simulink model "Schemi_Simulink_Tesina_Controlli"  (R2023b)
settings: Solver=VariableStepAuto  StartTime=0.0  StopTime=50  RelTol=1e-3
undefined symbols (not defined in the file): A, A_Kal, A_obs, Ar, B, B_Kal, B_obs, Br, C, C_Kal, C_obs, Cr, D, D_Kal, D_obs, Dr, Fi, Fr, Ki, Kr, Tc
libraries: simulink x7
settings Model: Creator=emman  LastModifiedBy=emman

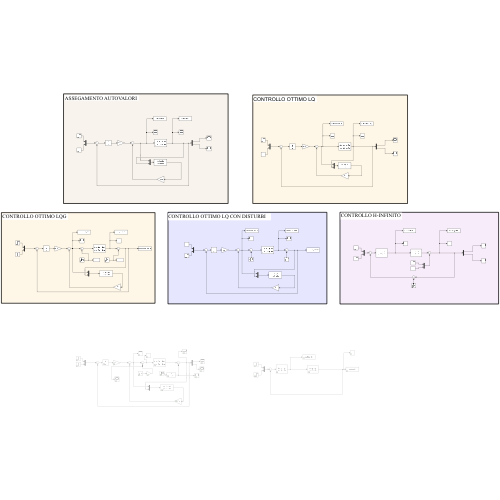
[thumbnail: Simulink's stored preview of the top-level diagram]
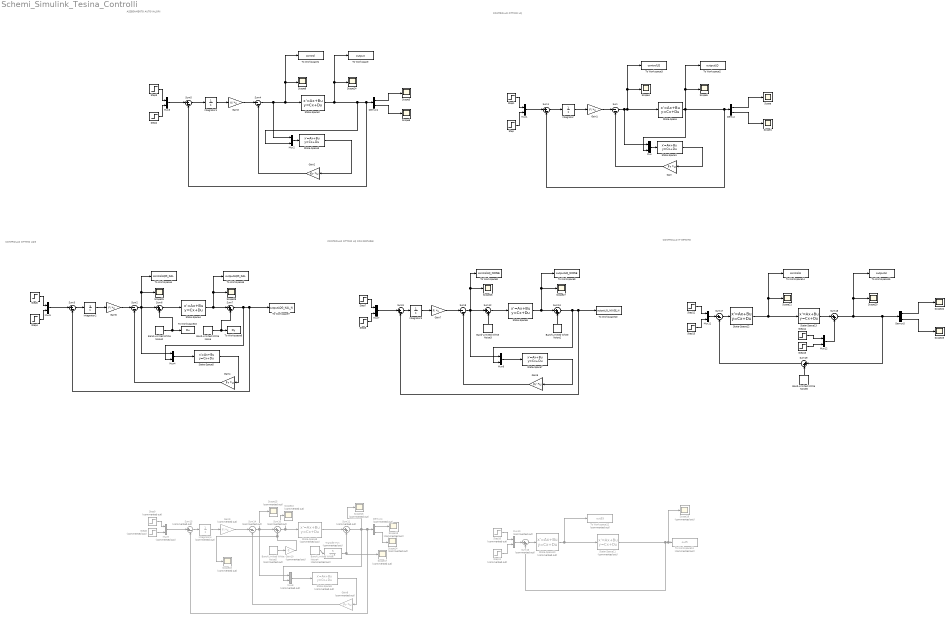
== system Schemi_Simulink_Tesina_Controlli ==
  note: CONTROLLO H-INFINITO
  note: CONTROLLO OTTIMO LQG
  note: CONTROLLO OTTIMO LQ CON DISTURBI
  note: CONTROLLO OTTIMO LQ
  note: ASSEGAMENTO AUTOVALORI
  Band-Limited White Noise : simulink/Sources/Band-Limited White Noise  Cov=NoisePower  Ts=Tc  seed=[23341]
  Band-Limited White Noise1 : simulink/Sources/Band-Limited White Noise  Cov=NoisePower  Ts=Tc  seed=[23341]
  Band-Limited White Noise2 : simulink/Sources/Band-Limited White Noise  Cov=Qnoise  Ts=Tc  seed=[23341]
  Band-Limited White Noise3 : simulink/Sources/Band-Limited White Noise  Cov=Qnoise  Ts=Tc  seed=[23341]
  Band-Limited White Noise4 : simulink/Sources/Band-Limited White Noise  Commented=on  Cov=NoisePower  Ts=Tc  seed=[23341]
  Band-Limited White Noise5 : simulink/Sources/Band-Limited White Noise  Commented=on  Cov=Qnoise  Ts=Tc  seed=[23341]
  Band-Limited White Noise6 : simulink/Sources/Band-Limited White Noise  Cov=NoisePower  Ts=Tc  seed=[23341]
  Demux : Demux  Outputs=2
  Demux1 : Demux  Outputs=2
  Demux4 : Demux  Commented=on  Outputs=2
  Demux5 : Demux  Outputs=2
  Gain : Gain  Gain=Fr  Multiplication=Matrix(K*u)
  Gain1 : Gain  Gain=Fi  Multiplication=Matrix(K*u)
  Gain10 : Gain  Commented=on  Gain=0
  Gain2 : Gain  Gain=Kr  Multiplication=Matrix(K*u)
  Gain3 : Gain  Gain=Ki  Multiplication=Matrix(K*u)
  Gain4 : Gain  Gain=Fr  Multiplication=Matrix(K*u)
  Gain5 : Gain  Gain=Fi  Multiplication=Matrix(K*u)
  Gain6 : Gain  Gain=Fr  Multiplication=Matrix(K*u)
  Gain7 : Gain  Gain=Fi  Multiplication=Matrix(K*u)
  Gain8 : Gain  Commented=on  Gain=Fr  Multiplication=Matrix(K*u)
  Gain9 : Gain  Commented=on  Gain=Fi  Multiplication=Matrix(K*u)
  Integrator{,1..3} (4 alike) : Integrator
  Integrator4 : Integrator  Commented=on
  Mux{,1..7,11..12} (10 alike) : Mux  Inputs=2
  Mux10 : Mux  Commented=on  Inputs=2
  Mux8 : Mux  Commented=on  Inputs=2
  Mux9 : Mux  Commented=on  Inputs=2
  Scope{,1,3..6,8,20..28} (16 alike) : Scope
  Scope{10,13..19} (8 alike) : Scope  Commented=on
  State-Space{,2,4,6} (4 alike) : StateSpace  A=A  B=B  C=C  D=D  InitialCondition=0  ParameterTunability=Unconstrained
  State-Space1 : StateSpace  A=A_obs  B=B_obs  C=C_obs  D=D_obs  InitialCondition=0
  State-Space10 : StateSpace  Commented=on  A=Ar  B=Br  C=Cr  D=Dr  InitialCondition=0
  State-Space11 : StateSpace  Commented=on  A=A  B=B  C=C  D=D  InitialCondition=0
  State-Space12 : StateSpace  A=Ar  B=Br  C=Cr  D=Dr  InitialCondition=0
  State-Space13 : StateSpace  A=A  B=B  C=C  D=D  InitialCondition=0
  State-Space3 : StateSpace  A=A_obs  B=B_obs  C=C_obs  D=D_obs  InitialCondition=0
  State-Space5 : StateSpace  A=A_Kal  B=B_Kal  C=C_Kal  D=D_Kal  InitialCondition=0
  State-Space7 : StateSpace  A=A_obs  B=B_obs  C=C_obs  D=D_obs  InitialCondition=0
  State-Space8 : StateSpace  Commented=on  A=A  B=B  C=C  D=D  InitialCondition=0  ParameterTunability=Unconstrained
  State-Space9 : StateSpace  Commented=on  A=A_obs  B=B_obs  C=C_obs  D=D_obs  InitialCondition=0
  Step{,2,4,6,13} (5 alike) : Step  Time=0  After=2.5  SampleTime=0
  Step{1,3,5,7,12} (5 alike) : Step  Time=0  After=2  SampleTime=0
  Step10 : Step  Commented=on  Time=0  After=2  SampleTime=0
  Step11 : Step  Commented=on  Time=0  After=2.5  SampleTime=0
  Step14 : Step  Time=0  After=0.5  SampleTime=0
  Step15 : Step  Time=0  After=0.5  SampleTime=0
  Step8 : Step  Commented=on  Time=0  After=2.5  SampleTime=0
  Step9 : Step  Commented=on  Time=0  After=2  SampleTime=0
  Sum{,2,4,8} (4 alike) : Sum  Inputs=|--
  Sum{1,3,5,9,17} (5 alike) : Sum  Inputs=|+-
  Sum10 : Sum  Commented=on  Inputs=|++
  Sum11 : Sum  Commented=on  Inputs=|++
  Sum{6..7,12..13,18..19} (6 alike) : Sum  Inputs=|++
  Sum14 : Sum  Commented=on  Inputs=|--
  Sum15 : Sum  Commented=on  Inputs=|+-
  Sum16 : Sum  Commented=on  Inputs=|+-
  To Workspace : ToWorkspace  VariableName=output  SaveFormat=Structure With Time  SampleTime=-1
  To Workspace1 : ToWorkspace  VariableName=control  SaveFormat=Structure With Time  SampleTime=-1
  To Workspace10 : ToWorkspace  VariableName=outputLQ_NOISE_N  SaveFormat=Structure With Time  SampleTime=-1
  To Workspace12 : ToWorkspace  Commented=on  VariableName=out55  SaveFormat=Structure With Time  SampleTime=-1
  To Workspace13 : ToWorkspace  Commented=on  VariableName=out5  SaveFormat=Structure With Time  SampleTime=-1
  To Workspace14 : ToWorkspace  VariableName=controlH  SaveFormat=Structure With Time  SampleTime=-1
  To Workspace15 : ToWorkspace  VariableName=outputH  SaveFormat=Structure With Time  SampleTime=-1
  To Workspace16 : ToWorkspace  VariableName=Du  SaveFormat=Structure With Time  SampleTime=-1
  To Workspace2 : ToWorkspace  VariableName=outputLQ  SaveFormat=Structure With Time  SampleTime=-1
  To Workspace3 : ToWorkspace  VariableName=controlLQ  SaveFormat=Structure With Time  SampleTime=-1
  To Workspace4 : ToWorkspace  VariableName=controlLQG_KAL  SaveFormat=Structure With Time  SampleTime=-1
  To Workspace5 : ToWorkspace  VariableName=outputLQG_KAL  SaveFormat=Structure With Time  SampleTime=-1
  To Workspace6 : ToWorkspace  VariableName=Dy  SaveFormat=Structure With Time  SampleTime=-1
  To Workspace7 : ToWorkspace  VariableName=outputLQG_KAL_N  SaveFormat=Structure With Time  SampleTime=-1
  To Workspace8 : ToWorkspace  VariableName=controlLQ_NOISE  SaveFormat=Structure With Time  SampleTime=-1
  To Workspace9 : ToWorkspace  VariableName=outputLQ_NOISE  SaveFormat=Structure With Time  SampleTime=-1
  Transfer Fcn : TransferFcn  Commented=on  Numerator=[5]  Denominator=[1 5]
  wires:
  Sum4/1 -> To Workspace1/1, Scope8/1, State-Space2/1, Mux2/1
  Integrator1/1 -> Gain3/1
  State-Space2/1 -> To Workspace/1, Scope24/1, Sum5/2, Demux1/1, Mux2/2
  State-Space3/1 -> Gain2/1
  Gain2/1 -> Sum4/2
  Demux1/1 -> Scope3/1
  Mux2/1 -> State-Space3/1
  Mux3/1 -> Sum5/1
  Demux1/2 -> Scope6/1
  Gain3/1 -> Sum4/1
  Step2/1 -> Mux3/2
  Sum5/1 -> Integrator1/1
  Step3/1 -> Mux3/1
  Gain1/1 -> Sum/1
  Sum/1 -> Scope4/1, To Workspace3/1, State-Space/1, Mux/1
  State-Space1/1 -> Gain/1
  Step/1 -> Mux1/2
  Mux1/1 -> Sum1/1
  Gain/1 -> Sum/2
  Sum1/1 -> Integrator/1
  State-Space/1 -> To Workspace2/1, Scope5/1, Sum1/2, Demux/1, Mux/2
  Step1/1 -> Mux1/1
  Mux/1 -> State-Space1/1
  Integrator/1 -> Gain1/1
  Demux/1 -> Scope/1
  Demux/2 -> Scope1/1
  Gain4/1 -> Sum2/2
  Step4/1 -> Mux5/2
  Sum3/1 -> Integrator2/1
  Step7/1 -> Mux7/1
  Integrator3/1 -> Gain7/1
  Sum8/1 -> Scope26/1, To Workspace8/1, Mux6/1, Sum12/1
  Sum2/1 -> Scope25/1, To Workspace4/1, Mux4/1, Sum6/1
  Band-Limited White Noise/1 -> Sum7/2, To Workspace6/1
  Sum6/1 -> State-Space4/1
  Band-Limited White Noise2/1 -> Sum6/2, To Workspace16/1
  Gain6/1 -> Sum8/2
  Band-Limited White Noise5/1 -> Gain10/1
  Gain10/1 -> Scope18/1, Sum10/2
  Sum14/1 -> Scope15/1, Mux8/1, Sum10/1
  State-Space8/1 -> Sum11/1
  Sum11/1 -> Scope16/1, Mux8/2, Sum15/2, Demux4/1
  Sum7/1 -> To Workspace7/1, Sum3/2, Mux4/2
  State-Space5/1 -> Gain4/1
  State-Space6/1 -> Scope27/1, To Workspace9/1, Sum13/1
  Gain5/1 -> Sum2/1
  Step8/1 -> Mux9/2
  Mux5/1 -> Sum3/1
  Gain8/1 -> Sum14/2
  Gain7/1 -> Sum8/1
  Gain9/1 -> Sum14/1
  Mux8/1 -> State-Space9/1
  Sum9/1 -> Integrator3/1
  Integrator2/1 -> Gain5/1
  Demux4/2 -> Scope14/1
  Mux9/1 -> Sum15/1
  Step9/1 -> Mux9/1
  Sum13/1 -> Mux6/2, To Workspace10/1, Sum9/2
  Band-Limited White Noise4/1 -> Transfer Fcn/1
  Integrator4/1 -> Gain9/1
  Mux6/1 -> State-Space7/1
  Transfer Fcn/1 -> Scope17/1, Sum11/2
  Sum12/1 -> State-Space6/1
  Sum10/1 -> Scope10/1, State-Space8/1
  Step6/1 -> Mux7/2
  State-Space9/1 -> Gain8/1
  Mux4/1 -> State-Space5/1
  Mux7/1 -> Sum9/1
  Sum15/1 -> Integrator4/1
  State-Space4/1 -> Scope28/1, To Workspace5/1, Sum7/1
  Step5/1 -> Mux5/1
  State-Space7/1 -> Gain6/1
  Demux4/1 -> Scope13/1
  Step12/1 -> Mux11/1
  Sum18/1 -> Sum19/1, Demux5/1, Scope20/1, To Workspace15/1
  State-Space13/1 -> Sum18/1
  Mux12/1 -> Sum18/2
  Sum17/1 -> State-Space12/1
  Step14/1 -> Mux12/1
  Mux11/1 -> Sum17/1
  Step11/1 -> Mux10/2
  Mux10/1 -> Sum16/1
  State-Space12/1 -> State-Space13/1, Scope21/1, To Workspace14/1
  Step15/1 -> Mux12/2
  State-Space11/1 -> Sum16/2, Scope19/1, To Workspace13/1
  Step13/1 -> Mux11/2
  Step10/1 -> Mux10/1
  Sum16/1 -> State-Space10/1
  State-Space10/1 -> State-Space11/1, To Workspace12/1
  Sum19/1 -> Sum17/2
  Band-Limited White Noise6/1 -> Sum19/2
  Demux5/1 -> Scope22/1
  Demux5/2 -> Scope23/1
  Band-Limited White Noise3/1 -> Sum12/2
  Band-Limited White Noise1/1 -> Sum13/2
